simulink model "ModelEx2"  (R2018b)
settings: Solver=ode4  StartTime=0.0  StopTime=10.0  FixedStep=0.01  RelTol=1e-3
values from neighbouring files (symbols this model uses):
  A = (1+(r/m))^(m)    (= 1.0304352292)    [SccriptEx3.m]    (also in ScriptEx2.m = [0 1 ;-I -N])
  Aprim = expm(h*A)    [ScriptEx2.m]
  B = [0 ;1]    [ScriptEx2.m]
  Bprim = double( int( expm( s*A )*B, s, 0, h ) )    [ScriptEx2.m]
  C = eye(2)    [ScriptEx2.m]
  Cprim = C    [ScriptEx2.m]
  D = [0 ;0]    [ScriptEx2.m]
  h = 0.4    [ScriptEx2.m]
  WPC = [-1.5, -1, -0.7, 0, 0.1, 1, 1.5]    [ScriptEx1.m]    (also in ScriptEx2.m = [1;-1])
settings Model: Creator=Joanna  LastModifiedBy=Joanna

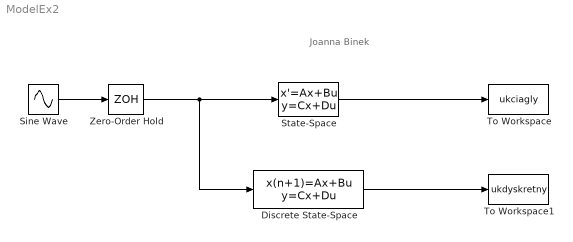
== system ModelEx2 ==
  note: Joanna Binek
  Discrete State-Space : DiscreteStateSpace  A=Aprim  B=Bprim  C=Cprim  D=D  InitialCondition=WPC  SampleTime=h
  Sine Wave : Sin  SampleTime=0
  State-Space : StateSpace  A=A  B=B  C=C  D=D  InitialCondition=WPC
  To Workspace : ToWorkspace  VariableName=ukciagly  SampleTime=-1
  To Workspace1 : ToWorkspace  VariableName=ukdyskretny  SampleTime=-1
  Zero-Order Hold : ZeroOrderHold  SampleTime=-1
  wires:
  Zero-Order Hold/1 -> Discrete State-Space/1, State-Space/1
  Sine Wave/1 -> Zero-Order Hold/1
  State-Space/1 -> To Workspace/1
  Discrete State-Space/1 -> To Workspace1/1
